simulink model "FinalModel"  (R2022a)
settings: Solver=VariableStepAuto  StartTime=0.0  StopTime=2  RelTol=1e-3
libraries: visionsources x2
settings Model: Creator=RAJSEKHAR  LastModifiedBy=RAJSEKHAR

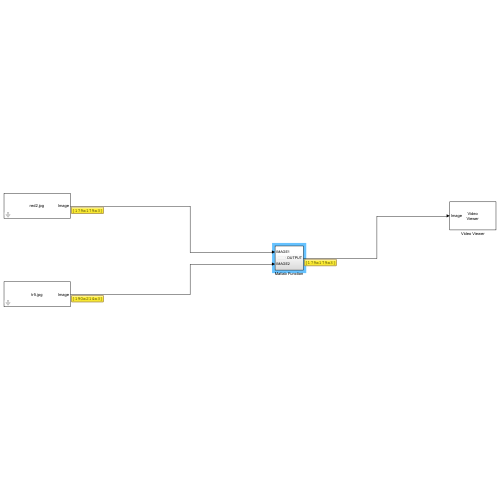
[thumbnail: Simulink's stored preview of the top-level diagram]
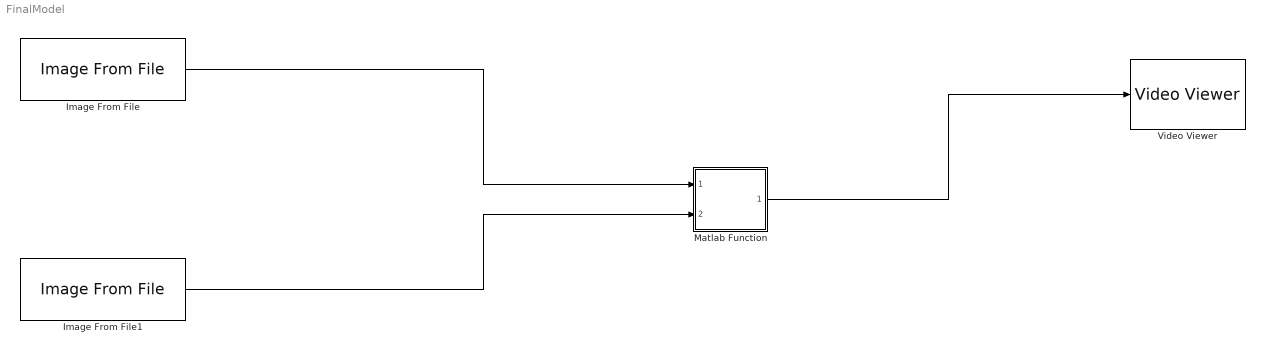
== system FinalModel ==
  Image From File : visionsources/Image From File  Tag=vipblks_nd  FileName=D:\Users\RAJSEKHAR\Downloads\red2.jpg  Ts=inf  imagePorts=One multidimensional signal  OutPortLabels=R|G|B  ImageDataType=Inherit from input image  sdImageDataType=uint(8)  Signed=on  WordLength=16  FractionLengthMode=User-defined  FractionLength=15
  Image From File1 : visionsources/Image From File  Tag=vipblks_nd  FileName=D:\Users\RAJSEKHAR\Downloads\tr5.jpg  Ts=inf  imagePorts=One multidimensional signal  OutPortLabels=R|G|B  ImageDataType=Inherit from input image  sdImageDataType=uint(8)  Signed=on  WordLength=16  FractionLengthMode=User-defined  FractionLength=15
  Matlab Function : Subsystem
  Video Viewer : VideoViewer  FigPos=[1376 608 418 304]
  wires:
  Matlab Function/1(OUTPUT) -> Video Viewer/1
  Image From File/1 -> Matlab Function/1(IMAGE1)
  Image From File1/1 -> Matlab Function/2(IMAGE2)

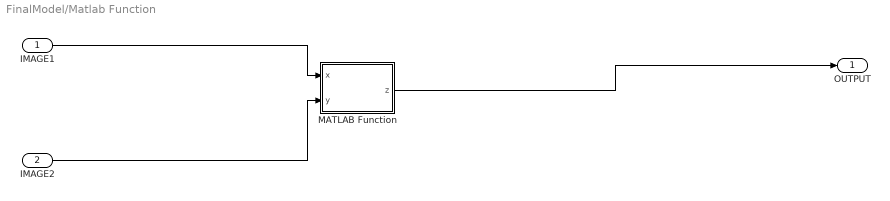
== system FinalModel/Matlab Function ==
  IMAGE1 : Inport
  IMAGE2 : Inport  Port=2
  MATLAB Function : MATLAB Function  TreatAsAtomicUnit=on
  OUTPUT : Outport
  wires:
  IMAGE2/1 -> MATLAB Function/2(y)
  IMAGE1/1 -> MATLAB Function/1(x)
  MATLAB Function/1(z) -> OUTPUT/1

== matlab function FinalModel/Matlab Function/MATLAB Function ==
  data: x input; z output; y input
function z = fcn(x, y)

%  clc
% clear
% close all
% warning off;
%  x=imread('D:\Users\RAJSEKHAR\Downloads\red2.jpg');
%  y=imread('D:\Users\RAJSEKHAR\Downloads\rect2.jpg');
g=size(x);
y=imresize(y,[g(1),g(2)]);
figure;
z=x-y;
pause(5);
